simulink model "kalman_test"  (R2021a)
settings: Solver=ode1  StartTime=0.0  StopTime=Tsim  RelTol=1e-3  EnableMultiTasking=on
values from neighbouring files (symbols this model uses):
  Ad = sys_d.A    [kalman_tuning.m]
  Bd = sys_d.B    [kalman_tuning.m]
  Cd = sys_d.C    [kalman_tuning.m]
  Kd = Kd'    [kalman_tuning.m]
  x0 = zeros(4,1)    [kalman_tuning.m]
settings Model: Creator=rbabuska  LastModifiedBy=chvan
settings SolverCC: AlgebraicLoopSolver=TrustRegion
settings DataIOCC: ExternalInput=ds  LimitDataPoints=on  LoadExternalInput=on  SaveFormat=Array  SignalLoggingSaveFormat=ModelDataLogs  ReturnWorkspaceOutputs=off
settings OptimizationCC: ExpressionDepthLimit=2147483647  LifeSpan=inf
settings DebuggingCC: UnderspecifiedInitializationDetection=Classic  MergeDetectMultiDrivingBlocksExec=none  FcnCallInpInsideContextMsg=warning  StateNameClashWarn=warning  SFUnexpectedBacktrackingDiag=warning  SFNoUnconditionalDefaultTransitionDiag=warning  SFExecutionAtInitializationDiag=none  SFMachineParentedDataDiag=warning  ArithmeticOperatorsInVariantConditions=warning
settings HardwareCC: ProdBitPerPointer=32  ProdBitPerSizeT=32  ProdBitPerPtrDiffT=32  ProdLargestAtomicFloat=None  ProdIntDivRoundTo=Undefined  ProdEndianess=Unspecified  ProdWordSize=32  ProdHWDeviceType=32-bit Generic
settings ModelReferenceCC: PropagateSignalLabelsOutOfModel=off
settings SFSimCC: SimUseLocalCustomCode=off  CustomCodeUndefinedFunction=UseInterfaceOnly
settings RTWCC: RTWUseLocalCustomCode=off
settings CodeAppCC: StateflowObjectComments=on
settings GRTTargetCC: TargetLangStandard=C89/C90 (ANSI)  CombineOutputUpdateFcns=off  GRTInterface=on
settings ConfigComp: CovMetricSettings=dw  CovSaveCumulativeToWorkspaceVar=on  CovSaveSingleToWorkspaceVar=on  CovExternalEMLEnable=off  CovSFcnEnable=off

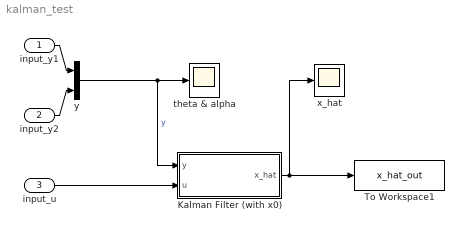
== system kalman_test ==
  input_y1 : Inport
  input_y2 : Inport  Port=2
  input_u : Inport  Port=3
  Kalman Filter (with x0) : Subsystem
  To Workspace1 : ToWorkspace  VariableName=x_hat_out  SaveFormat=Timeseries  SampleTime=-1
  theta & alpha : Scope
  x_hat : Scope
  y : Concatenate
  wires:
  y/1 -> theta & alpha/1, Kalman Filter (with x0)/1(y)  "y"
  Kalman Filter (with x0)/1(x_hat) -> x_hat/1, To Workspace1/1
  input_y2/1 -> y/2
  input_y1/1 -> y/1
  input_u/1 -> Kalman Filter (with x0)/2(u)

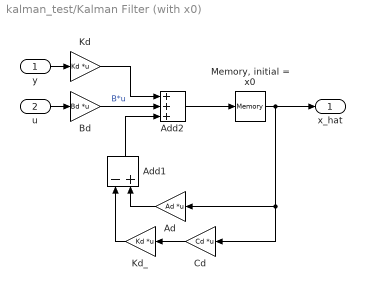
== system kalman_test/Kalman Filter (with x0) ==
  y : Inport
  u : Inport  Port=2
  Ad : Gain  Gain=Ad  Multiplication=Matrix(K*u) (u vector)
  Add1 : Sum  Inputs=-+
  Add2 : Sum  Inputs=+++
  Bd : Gain  Gain=Bd  Multiplication=Matrix(K*u) (u vector)
  Cd : Gain  Gain=Cd  Multiplication=Matrix(K*u) (u vector)
  Kd : Gain  Gain=Kd  Multiplication=Matrix(K*u) (u vector)
  Kd_ : Gain  Gain=Kd  Multiplication=Matrix(K*u) (u vector)
  "Memory, initial = x0" : Memory  InitialCondition=x0
  x_hat : Outport
  wires:
  Add1/1 -> Add2/3
  Ad/1 -> Add1/2
  Bd/1 -> Add2/2  "B*u"
  Kd_/1 -> Add1/1
  Kd/1 -> Add2/1
  Cd/1 -> Kd_/1
  y/1 -> Kd/1
  u/1 -> Bd/1
  Add2/1 -> "Memory, initial = x0"/1
  "Memory, initial = x0"/1 -> Cd/1, Ad/1, x_hat/1
